simulink model "Caster_4_Whl_Hill"  (R2026a)
settings: Solver=ode23t  StopTime=2.5  FixedStep=1e-3  MaxStep=0.01  RelTol=1e-4  AbsTol=1e-5  EnableMultiTasking=on
StartFcn:
  | tic;
StopFcn:
  | Elapsed_Sim_Time = toc;
  | disp(['Elapsed Sim Time = ' num2str(Elapsed_Sim_Time)]);
model workspace (MATLAB code in the model file):
  | whl.rad = 0.02;
  | whl.thickness = 0.005;
  | 
  | axle.length = 0.2;
  | axle.radius = 0.005;
  | platform.width = 0.1;
  | platform.length = 0.15;
  | platform.thickness = 0.005;
  | platform.offset = 0.05;
  | 
  | caster_axis.rad = 0.005;
  | caster_axis.length = 0.03;
  | 
  | bumper.rad = platform.offset+whl.rad;
  | 
  | 
  | 
  | table.length = 0.5;
  | table.thickness = 0.01;
  | tableWhl.contact.k = 1e3;
  | tableWhl.contact.b = 1e2;
  | 
  | steel.density = 8000; %kg/m^3
  | 
  | start_pos.x = -0.2;
  | start_pos.y = 0.2;
  | 
  | l_whl_trq = [0 0 0 0.5 0 0 0 -0.5 1.0 0 0 0 -1.0 0.5 0 0 0 -0.5 -1.5 0 0 0 1.5].'*0.00005;
  | r_whl_trq = [0 0 0 2.0 0 0 0 -2.0 1.0 0 0 0 -1.0 1.0 0 0 0 -1.0 -1.5 0 0 0 1.5].'*0.00005;
  | 
  | l_whl_trq = [-0.45 0 -0.1 0 0]*7.5e-5*100;
  | r_whl_trq = [-0.45 0 -0.1 0 0]*7.5e-5*100;
  | 
  | muk = 0.7;
  | mus = 0.5;
  | vth =1e-2;
  | 
  | % Floor dimensions
  | flr1_len = 1;
  | flr1_wid = 0.5;
  | flr1_dep = 0.01;
  | flr1_ang = 0;  % deg, rel to world
  | 
  | flr2_len = flr1_len/8;
  | flr2_wid = flr1_wid;
  | flr2_dep = flr1_dep;
  | flr2_ang = 10; % deg, rel to World
  | 
  | flr3_len = flr1_len/3;
  | flr3_wid = flr1_wid;
  | flr3_dep = flr1_dep;
  | flr3_ang = 0;  % deg, rel to World
  | 
  | % Visualize Surfaces
  | flr_dep_pcnt = 0.1;  %(0-1)
  | flr_clr = [1 1 1]*0.95;
undefined symbols (not defined in the file or in its folder): X, Y, Z
libraries: sm_lib x43, Contact_Forces_Lib x16, nesl_utility x5, Parts_Lib x4, simulink x2
(part 2 of 2)

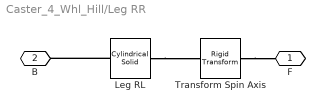
== system Caster_4_Whl_Hill/Leg RR ==
  Leg RL : sm_lib/Body Elements/Cylindrical Solid  CylinderRadius=caster_axis.rad  CylinderRadiusUnits=m  CylinderLength=caster_axis.length  CylinderLengthUnits=m  ExportEntireGeometry=off  InertiaType=CalculateFromGeometry  BasedOnType=Density  Density=1000  DensityUnits=kg/m^3  Mass=1  MassUnits=kg  CenterOfMass=[0 0 0]  CenterOfMassUnits=m  MomentsOfInertia=[1 1 1]  MomentsOfInertiaUnits=kg*m^2  ProductsOfInertia=[0 0 0]  ProductsOfInertiaUnits=kg*m^2  GraphicType=FromGeometry  MarkerShape=Sphere  MarkerSize=10  GraphicVisPropType=SimpleVisualProperties  GraphicDiffuseColor=[0.5 0.5 0.5]  GraphicOpacity=1.0  GraphicSpecularColor=[0.5 0.5 0.5 1.0]  GraphicAmbientColor=[0.15 0.15 0.15 1.0]  GraphicEmissiveColor=[0.0 0.0 0.0 1.0]  GraphicShininess=75  DoExposeReferenceFrame=off  SerializedFrames=<Frames><Frame><Id>Frame1</Id><Value><Name>B</Name><Origin><Source>GeometricFeature</Source><FeatureName>top surface</FeatureName></Origin><PrimaryAxis><DefinedDirection>+Z</DefinedDirection><Source>ReferenceFrame</Source><SourceDirection>+Z</SourceDirection><FeatureName></FeatureName></PrimaryAxis><SecondaryAxis><DefinedDirection>+X</DefinedDirection><Source>ReferenceFrame</Source><SourceDirection>+X</SourceDirection><FeatureName></FeatureName></SecondaryAxis></Value></Frame><Frame><Id>Frame2</Id><Value><Name>F</Name><Origin><Source>GeometricFeature</Source><FeatureName>bottom surface</FeatureName></Origin><PrimaryAxis><DefinedDirection>+Z</DefinedDirection><Source>ReferenceFrame</Source><SourceDirection>+Z</SourceDirection><FeatureName></FeatureName></PrimaryAxis><SecondaryAxis><DefinedDirection>+X</DefinedDirection><Source>ReferenceFrame</Source><SourceDirection>+X</SourceDirection><FeatureName></FeatureName></SecondaryAxis></Value></Frame></Frames>
  Transform Spin Axis : sm_lib/Frames and Transforms/Rigid Transform  RotationMethod=StandardAxis  FollAlignAxisA=+X  BaseAlignAxisA=+Y  FollAlignAxisB=+Y  BaseAlignAxisB=+Z  RotationStandardAxis=+X  RotationAngle=-90  RotationAngleUnits=deg  RotationArbitraryAxis=[0 0 1]  RotationSequenceAxes=FollowerAxes  RotationSequence=XYX  RotationSequenceAngles=[0 0 0]  RotationSequenceAnglesUnits=deg  RotationMatrix=[1 0 0; 0 1 0; 0 0 1]  Quaternion=[1 0 0 0]  TranslationMethod=None  TranslationCartesianOffset=[0 0 0]  TranslationCartesianOffsetUnits=m  TranslationStandardAxis=+Z  TranslationStandardOffset=0  TranslationStandardOffsetUnits=m  TranslationROffset=0  TranslationROffsetUnits=m  TranslationThetaOffset=0  TranslationThetaOffsetUnits=deg  TranslationZOffset=0  TranslationZOffsetUnits=m
  F : PMIOPort  Side=Right
  B : PMIOPort  Port=2  Side=Left
  connections:
  Leg RL/RConn1 -- Transform Spin Axis/LConn1
  Transform Spin Axis/RConn1 -- F/RConn1
  Leg RL/LConn1 -- B/RConn1

== system Caster_4_Whl_Hill/MotorL ==
  Rate Transition : RateTransition
  Repeating Sequence Stair : simulink/Sources/Repeating Sequence Stair  OutValues=l_whl_trq  tsamp=0.7  OutMin=[]  OutMax=[]  OutDataTypeStr=double  OutputDataTypeScalingMode=double  OutDataType=fixdt(0,8)  ConRadixGroup=Best Precision: Vector-wise  OutScaling=2^-12
  Simulink-PS Converter1 : nesl_utility/Simulink-PS Converter  PhysicalDomain=network_engine_domain  SubClassName=ps_input  LeftPortType=input  RightPortType=output  PseudoPeriodic=off  Frequencies=[]  NoiseDistribution=none  NoiseParameters=[]  Unit=1  AffineConversion=off  FilteringAndDerivatives=filter  SimscapeFilterOrder=2  InputFilterTimeConstant=0.005  UdotUserProvided=1
  trq : PMIOPort  Side=Right
  wires:
  Repeating Sequence Stair/1 -> Rate Transition/1
  Rate Transition/1 -> Simulink-PS Converter1/1
  connections:
  trq/RConn1 -- Simulink-PS Converter1/RConn1

== system Caster_4_Whl_Hill/MotorR ==
  Rate Transition : RateTransition
  Repeating Sequence Stair : simulink/Sources/Repeating Sequence Stair  OutValues=r_whl_trq  tsamp=0.7  OutMin=[]  OutMax=[]  OutDataTypeStr=double  OutputDataTypeScalingMode=double  OutDataType=fixdt(0,8)  ConRadixGroup=Best Precision: Vector-wise  OutScaling=2^-12
  Simulink-PS Converter : nesl_utility/Simulink-PS Converter  PhysicalDomain=network_engine_domain  SubClassName=ps_input  LeftPortType=input  RightPortType=output  PseudoPeriodic=off  Frequencies=[]  NoiseDistribution=none  NoiseParameters=[]  Unit=1  AffineConversion=off  FilteringAndDerivatives=filter  SimscapeFilterOrder=2  InputFilterTimeConstant=0.005  UdotUserProvided=1
  trq : PMIOPort  Side=Right
  wires:
  Repeating Sequence Stair/1 -> Rate Transition/1
  Rate Transition/1 -> Simulink-PS Converter/1
  connections:
  Simulink-PS Converter/RConn1 -- trq/RConn1

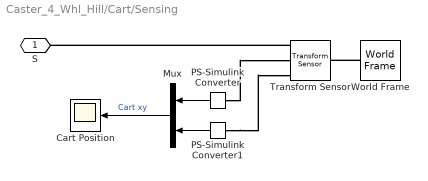
== system Caster_4_Whl_Hill/Cart/Sensing ==
  Cart Position : Scope
      settings: ActiveDisplayYMinimum=-0.86321  ActiveDisplayYMaximum=0.10356  DataLoggingSaveFormat=Array
  Mux : Mux  Inputs=2
  PS-Simulink Converter : nesl_utility/PS-Simulink Converter  PhysicalDomain=network_engine_domain  SubClassName=ps_output  LeftPortType=input  RightPortType=output  PseudoPeriodic=off  Frequencies=[]  VectorFormat=1-D array  Unit=m  AffineConversion=off
  PS-Simulink Converter1 : nesl_utility/PS-Simulink Converter  PhysicalDomain=network_engine_domain  SubClassName=ps_output  LeftPortType=input  RightPortType=output  PseudoPeriodic=off  Frequencies=[]  VectorFormat=1-D array  Unit=m  AffineConversion=off
  Transform Sensor : sm_lib/Frames and Transforms/Transform Sensor  MeasurementFrame=World  RotationSequence=XYX  SenseAngle=off  SenseAxis=off  SenseQ=off  SenseR=off  SenseRotationSequence=off  SenseOmegaX=off  SenseOmegaY=off  SenseOmegaZ=off  SenseOmega=off  SenseQDot=off  SenseRDot=off  SenseRotationSequenceDot=off  SenseAlphaX=off  SenseAlphaY=off  SenseAlphaZ=off  SenseAlpha=off  SenseQDDot=off  SenseRDDot=off  SenseX=on  SenseY=off  SenseZ=on  SenseXYZ=off  SenseRad=off  SenseAzim=off  SenseDist=off  SenseInc=off  SenseXDot=off  SenseYDot=off  SenseZDot=off  SenseXYZDot=off  SenseRadDot=off  SenseAzimDot=off  SenseDistDot=off  SenseIncDot=off  SenseXDDot=off  SenseYDDot=off  SenseZDDot=off  SenseXYZDDot=off  SenseRadDDot=off  SenseAzimDDot=off  SenseDistDDot=off  SenseIncDDot=off
  World Frame : sm_lib/Frames and Transforms/World Frame
  S : PMIOPort  Side=Left
  wires:
  PS-Simulink Converter/1 -> Mux/1
  PS-Simulink Converter1/1 -> Mux/2
  Mux/1 -> Cart Position/1  "Cart xy"
  connections:
  PS-Simulink Converter/LConn1 -- Transform Sensor/RConn2
  World Frame/RConn1 -- Transform Sensor/LConn1
  Transform Sensor/RConn1 -- S/RConn1
  PS-Simulink Converter1/LConn1 -- Transform Sensor/RConn3

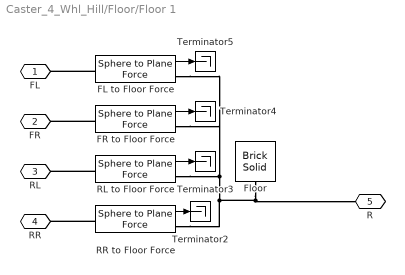
== system Caster_4_Whl_Hill/Floor/Floor 1 ==
  FL to Floor Force : Contact_Forces_Lib/3D/Sphere to Plane Force  sphere_rad=whl.rad  plane_lenx=flr1_len  plane_leny=flr1_wid  plane_depth=flr1_dep/2  force_law=Linear  k_contact=tableWhl.contact.k  b_contact=tableWhl.contact.b  pen_full_damp_F=1e-4  pen_exponent=1  custom_param_1=1  custom_param_2=1  friction_law=Stick-Slip Continuous  mu_kinetic=muk  mu_static=mus  v_thr=vth  vis_on=off  vis_opc_en=0  vis_len_plaBz=flr1_dep*flr_dep_pcnt  vis_clr=[0.9 0.2 0.2]  vis_opc=0.7
  FR to Floor Force : Contact_Forces_Lib/3D/Sphere to Plane Force  sphere_rad=whl.rad  plane_lenx=flr1_len  plane_leny=flr1_wid  plane_depth=flr1_dep/2  force_law=Linear  k_contact=tableWhl.contact.k  b_contact=tableWhl.contact.b  pen_full_damp_F=1e-4  pen_exponent=1  custom_param_1=1  custom_param_2=1  friction_law=Stick-Slip Continuous  mu_kinetic=muk  mu_static=mus  v_thr=vth  vis_on=off  vis_opc_en=0  vis_len_plaBz=flr1_dep*flr_dep_pcnt  vis_clr=[0.9 0.2 0.2]  vis_opc=0.7
  Floor : sm_lib/Body Elements/Brick Solid  BrickDimensions=[flr1_len flr1_wid flr1_dep]  BrickDimensionsUnits=m  ExportEntireGeometry=off  InertiaType=CalculateFromGeometry  BasedOnType=Density  Density=1000  DensityUnits=kg/m^3  Mass=1  MassUnits=kg  CenterOfMass=[0 0 0]  CenterOfMassUnits=m  MomentsOfInertia=[1 1 1]  MomentsOfInertiaUnits=kg*m^2  ProductsOfInertia=[0 0 0]  ProductsOfInertiaUnits=kg*m^2  GraphicType=FromGeometry  MarkerShape=Sphere  MarkerSize=10  GraphicVisPropType=SimpleVisualProperties  GraphicDiffuseColor=flr_clr  GraphicOpacity=1.0  GraphicSpecularColor=[0.5 0.5 0.5 1.0]  GraphicAmbientColor=[0.15 0.15 0.15 1.0]  GraphicEmissiveColor=[0.0 0.0 0.0 1.0]  GraphicShininess=75  DoExposeReferenceFrame=on  SerializedFrames=<Frames/>
  RL to Floor Force : Contact_Forces_Lib/3D/Sphere to Plane Force  sphere_rad=whl.rad  plane_lenx=flr1_len  plane_leny=flr1_wid  plane_depth=flr1_dep/2  force_law=Linear  k_contact=tableWhl.contact.k  b_contact=tableWhl.contact.b  pen_full_damp_F=1e-4  pen_exponent=1  custom_param_1=1  custom_param_2=1  friction_law=Stick-Slip Continuous  mu_kinetic=muk  mu_static=mus  v_thr=vth  vis_on=off  vis_opc_en=0  vis_len_plaBz=flr1_dep*flr_dep_pcnt  vis_clr=[0.9 0.2 0.2]  vis_opc=0.7
  RR to Floor Force : Contact_Forces_Lib/3D/Sphere to Plane Force  sphere_rad=whl.rad  plane_lenx=flr1_len  plane_leny=flr1_wid  plane_depth=flr1_dep/2  force_law=Linear  k_contact=tableWhl.contact.k  b_contact=tableWhl.contact.b  pen_full_damp_F=1e-4  pen_exponent=1  custom_param_1=1  custom_param_2=1  friction_law=Stick-Slip Continuous  mu_kinetic=muk  mu_static=mus  v_thr=vth  vis_on=off  vis_opc_en=0  vis_len_plaBz=flr1_dep*flr_dep_pcnt  vis_clr=[0.9 0.2 0.2]  vis_opc=0.7
  Terminator{2..5} (4 alike) : Terminator
  FL : PMIOPort  Side=Left
  FR : PMIOPort  Port=2  Side=Left
  RL : PMIOPort  Port=3  Side=Left
  RR : PMIOPort  Port=4  Side=Left
  R : PMIOPort  Port=5  Side=Right
  wires:
  FR to Floor Force/1 -> Terminator4/1
  FL to Floor Force/1 -> Terminator5/1
  RL to Floor Force/1 -> Terminator3/1
  RR to Floor Force/1 -> Terminator2/1
  connections:
  Floor/RConn1 -- R/RConn1 -- RR to Floor Force/RConn1 -- RL to Floor Force/RConn1 -- FR to Floor Force/RConn1 -- FL to Floor Force/RConn1
  FR to Floor Force/LConn1 -- FR/RConn1
  RR to Floor Force/LConn1 -- RR/RConn1
  RL to Floor Force/LConn1 -- RL/RConn1
  FL to Floor Force/LConn1 -- FL/RConn1

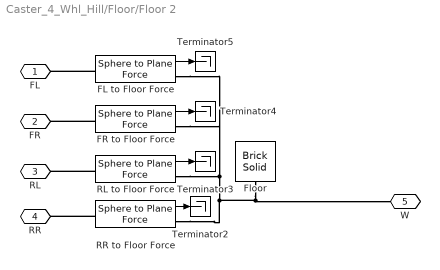
== system Caster_4_Whl_Hill/Floor/Floor 2 ==
  FL to Floor Force : Contact_Forces_Lib/3D/Sphere to Plane Force  sphere_rad=whl.rad  plane_lenx=flr2_len  plane_leny=flr2_wid  plane_depth=flr2_dep/2  force_law=Linear  k_contact=tableWhl.contact.k  b_contact=tableWhl.contact.b  pen_full_damp_F=1e-4  pen_exponent=1  custom_param_1=1  custom_param_2=1  friction_law=Stick-Slip Continuous  mu_kinetic=muk  mu_static=mus  v_thr=vth  vis_on=off  vis_opc_en=0  vis_len_plaBz=flr2_dep*flr_dep_pcnt  vis_clr=[0.9 0.2 0.2]  vis_opc=0.7
  FR to Floor Force : Contact_Forces_Lib/3D/Sphere to Plane Force  sphere_rad=whl.rad  plane_lenx=flr2_len  plane_leny=flr2_wid  plane_depth=flr2_dep/2  force_law=Linear  k_contact=tableWhl.contact.k  b_contact=tableWhl.contact.b  pen_full_damp_F=1e-4  pen_exponent=1  custom_param_1=1  custom_param_2=1  friction_law=Stick-Slip Continuous  mu_kinetic=muk  mu_static=mus  v_thr=vth  vis_on=off  vis_opc_en=0  vis_len_plaBz=flr2_dep*flr_dep_pcnt  vis_clr=[0.9 0.2 0.2]  vis_opc=0.7
  Floor : sm_lib/Body Elements/Brick Solid  BrickDimensions=[flr2_len flr2_wid flr2_dep]  BrickDimensionsUnits=m  ExportEntireGeometry=off  InertiaType=CalculateFromGeometry  BasedOnType=Density  Density=1000  DensityUnits=kg/m^3  Mass=1  MassUnits=kg  CenterOfMass=[0 0 0]  CenterOfMassUnits=m  MomentsOfInertia=[1 1 1]  MomentsOfInertiaUnits=kg*m^2  ProductsOfInertia=[0 0 0]  ProductsOfInertiaUnits=kg*m^2  GraphicType=FromGeometry  MarkerShape=Sphere  MarkerSize=10  GraphicVisPropType=SimpleVisualProperties  GraphicDiffuseColor=flr_clr  GraphicOpacity=1.0  GraphicSpecularColor=[0.5 0.5 0.5 1.0]  GraphicAmbientColor=[0.15 0.15 0.15 1.0]  GraphicEmissiveColor=[0.0 0.0 0.0 1.0]  GraphicShininess=75  DoExposeReferenceFrame=on  SerializedFrames=<Frames/>
  RL to Floor Force : Contact_Forces_Lib/3D/Sphere to Plane Force  sphere_rad=whl.rad  plane_lenx=flr2_len  plane_leny=flr2_wid  plane_depth=flr2_dep/2  force_law=Linear  k_contact=tableWhl.contact.k  b_contact=tableWhl.contact.b  pen_full_damp_F=1e-4  pen_exponent=1  custom_param_1=1  custom_param_2=1  friction_law=Stick-Slip Continuous  mu_kinetic=muk  mu_static=mus  v_thr=vth  vis_on=off  vis_opc_en=0  vis_len_plaBz=flr2_dep*flr_dep_pcnt  vis_clr=[0.9 0.2 0.2]  vis_opc=0.7
  RR to Floor Force : Contact_Forces_Lib/3D/Sphere to Plane Force  sphere_rad=whl.rad  plane_lenx=flr2_len  plane_leny=flr2_wid  plane_depth=flr2_dep/2  force_law=Linear  k_contact=tableWhl.contact.k  b_contact=tableWhl.contact.b  pen_full_damp_F=1e-4  pen_exponent=1  custom_param_1=1  custom_param_2=1  friction_law=Stick-Slip Continuous  mu_kinetic=muk  mu_static=mus  v_thr=vth  vis_on=off  vis_opc_en=0  vis_len_plaBz=flr2_dep*flr_dep_pcnt  vis_clr=[0.9 0.2 0.2]  vis_opc=0.7
  Terminator{2..5} (4 alike) : Terminator
  FL : PMIOPort  Side=Left
  FR : PMIOPort  Port=2  Side=Left
  RL : PMIOPort  Port=3  Side=Left
  RR : PMIOPort  Port=4  Side=Left
  W : PMIOPort  Port=5  Side=Right
  wires:
  RR to Floor Force/1 -> Terminator2/1
  RL to Floor Force/1 -> Terminator3/1
  FL to Floor Force/1 -> Terminator5/1
  FR to Floor Force/1 -> Terminator4/1
  connections:
  FL to Floor Force/LConn1 -- FL/RConn1
  RL to Floor Force/LConn1 -- RL/RConn1
  RR to Floor Force/LConn1 -- RR/RConn1
  FR to Floor Force/LConn1 -- FR/RConn1
  Floor/RConn1 -- W/RConn1 -- RR to Floor Force/RConn1 -- FL to Floor Force/RConn1 -- FR to Floor Force/RConn1 -- RL to Floor Force/RConn1

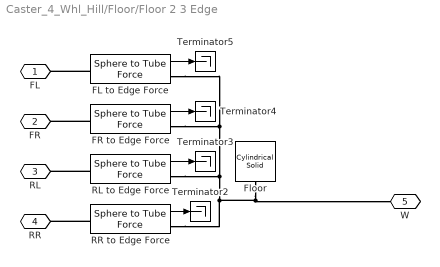
== system Caster_4_Whl_Hill/Floor/Floor 2 3 Edge ==
  FL to Edge Force : Contact_Forces_Lib/3D/Sphere to Tube Force  radius_sphere=whl.rad  radius_tube=flr2_dep/2*(1-0.1)  d_tube=flr2_dep/2*(2*0.1)  l_tube=flr2_wid  active_angle=[-flr2_ang 0]  force_law=Linear  k_contact=tableWhl.contact.k  b_contact=tableWhl.contact.b  pen_full_damp_F=1e-4  pen_exponent=1  custom_param_1=1  custom_param_2=1  friction_law=Stick-Slip Continuous  mu_kinetic=muk  mu_static=mus  v_thr=vth  vis_on=off  vis_opc_en=0  vis_len_tubBx=flr2_dep*flr_dep_pcnt  vis_clr=[0.9 0.2 0.2]  vis_opc=0.7
      settings: SourceProductName=Simscape Multibody Contact Forces Library
  FR to Edge Force : Contact_Forces_Lib/3D/Sphere to Tube Force  radius_sphere=whl.rad  radius_tube=flr2_dep/2*(1-0.1)  d_tube=flr2_dep/2*(2*0.1)  l_tube=flr2_wid  active_angle=[-flr2_ang 0]  force_law=Linear  k_contact=tableWhl.contact.k  b_contact=tableWhl.contact.b  pen_full_damp_F=1e-4  pen_exponent=1  custom_param_1=1  custom_param_2=1  friction_law=Stick-Slip Continuous  mu_kinetic=muk  mu_static=mus  v_thr=vth  vis_on=off  vis_opc_en=0  vis_len_tubBx=flr2_dep*flr_dep_pcnt  vis_clr=[0.9 0.2 0.2]  vis_opc=0.7
      settings: SourceProductName=Simscape Multibody Contact Forces Library
  Floor : sm_lib/Body Elements/Cylindrical Solid  CylinderRadius=flr2_dep/2  CylinderRadiusUnits=m  CylinderLength=flr2_wid  CylinderLengthUnits=m  ExportEntireGeometry=off  InertiaType=CalculateFromGeometry  BasedOnType=Density  Density=1000  DensityUnits=kg/m^3  Mass=1  MassUnits=kg  CenterOfMass=[0 0 0]  CenterOfMassUnits=m  MomentsOfInertia=[1 1 1]  MomentsOfInertiaUnits=kg*m^2  ProductsOfInertia=[0 0 0]  ProductsOfInertiaUnits=kg*m^2  GraphicType=FromGeometry  MarkerShape=Sphere  MarkerSize=10  GraphicVisPropType=SimpleVisualProperties  GraphicDiffuseColor=flr_clr  GraphicOpacity=1.0  GraphicSpecularColor=[0.5 0.5 0.5 1.0]  GraphicAmbientColor=[0.15 0.15 0.15 1.0]  GraphicEmissiveColor=[0.0 0.0 0.0 1.0]  GraphicShininess=75  DoExposeReferenceFrame=on  SerializedFrames=<Frames/>
  RL to Edge Force : Contact_Forces_Lib/3D/Sphere to Tube Force  radius_sphere=whl.rad  radius_tube=flr2_dep/2*(1-0.1)  d_tube=flr2_dep/2*(2*0.1)  l_tube=flr2_wid  active_angle=[-flr2_ang 0]  force_law=Linear  k_contact=tableWhl.contact.k  b_contact=tableWhl.contact.b  pen_full_damp_F=1e-4  pen_exponent=1  custom_param_1=1  custom_param_2=1  friction_law=Stick-Slip Continuous  mu_kinetic=muk  mu_static=mus  v_thr=vth  vis_on=off  vis_opc_en=0  vis_len_tubBx=flr2_dep*flr_dep_pcnt  vis_clr=[0.9 0.2 0.2]  vis_opc=0.7
      settings: SourceProductName=Simscape Multibody Contact Forces Library
  RR to Edge Force : Contact_Forces_Lib/3D/Sphere to Tube Force  radius_sphere=whl.rad  radius_tube=flr2_dep/2*(1-0.1)  d_tube=flr2_dep/2*(2*0.1)  l_tube=flr2_wid  active_angle=[-flr2_ang 0]  force_law=Linear  k_contact=tableWhl.contact.k  b_contact=tableWhl.contact.b  pen_full_damp_F=1e-4  pen_exponent=1  custom_param_1=1  custom_param_2=1  friction_law=Stick-Slip Continuous  mu_kinetic=muk  mu_static=mus  v_thr=vth  vis_on=off  vis_opc_en=0  vis_len_tubBx=flr2_dep*flr_dep_pcnt  vis_clr=[0.9 0.2 0.2]  vis_opc=0.7
      settings: SourceProductName=Simscape Multibody Contact Forces Library
  Terminator{2..5} (4 alike) : Terminator
  FL : PMIOPort  Side=Left
  FR : PMIOPort  Port=2  Side=Left
  RL : PMIOPort  Port=3  Side=Left
  RR : PMIOPort  Port=4  Side=Left
  W : PMIOPort  Port=5  Side=Right
  wires:
  FR to Edge Force/1 -> Terminator4/1
  FL to Edge Force/1 -> Terminator5/1
  RL to Edge Force/1 -> Terminator3/1
  RR to Edge Force/1 -> Terminator2/1
  connections:
  RL to Edge Force/RConn1 -- FR to Edge Force/RConn1 -- FL to Edge Force/RConn1 -- RR to Edge Force/RConn1 -- W/RConn1 -- Floor/RConn1
  FR to Edge Force/LConn1 -- FR/RConn1
  RR to Edge Force/LConn1 -- RR/RConn1
  RL to Edge Force/LConn1 -- RL/RConn1
  FL to Edge Force/LConn1 -- FL/RConn1

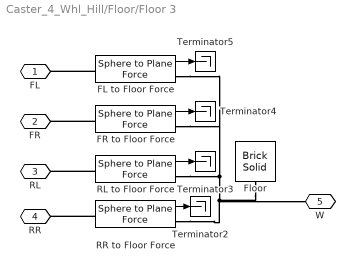
== system Caster_4_Whl_Hill/Floor/Floor 3 ==
  FL to Floor Force : Contact_Forces_Lib/3D/Sphere to Plane Force  sphere_rad=whl.rad  plane_lenx=flr3_len  plane_leny=flr3_wid  plane_depth=flr3_dep/2  force_law=Linear  k_contact=tableWhl.contact.k  b_contact=tableWhl.contact.b  pen_full_damp_F=1e-4  pen_exponent=1  custom_param_1=1  custom_param_2=1  friction_law=Stick-Slip Continuous  mu_kinetic=muk  mu_static=mus  v_thr=vth  vis_on=off  vis_opc_en=0  vis_len_plaBz=flr3_dep*flr_dep_pcnt  vis_clr=[0.9 0.2 0.2]  vis_opc=0.7
  FR to Floor Force : Contact_Forces_Lib/3D/Sphere to Plane Force  sphere_rad=whl.rad  plane_lenx=flr3_len  plane_leny=flr3_wid  plane_depth=flr3_dep/2  force_law=Linear  k_contact=tableWhl.contact.k  b_contact=tableWhl.contact.b  pen_full_damp_F=1e-4  pen_exponent=1  custom_param_1=1  custom_param_2=1  friction_law=Stick-Slip Continuous  mu_kinetic=muk  mu_static=mus  v_thr=vth  vis_on=off  vis_opc_en=0  vis_len_plaBz=flr3_dep*flr_dep_pcnt  vis_clr=[0.9 0.2 0.2]  vis_opc=0.7
  Floor : sm_lib/Body Elements/Brick Solid  BrickDimensions=[flr3_len flr3_wid flr3_dep]  BrickDimensionsUnits=m  ExportEntireGeometry=off  InertiaType=CalculateFromGeometry  BasedOnType=Density  Density=1000  DensityUnits=kg/m^3  Mass=1  MassUnits=kg  CenterOfMass=[0 0 0]  CenterOfMassUnits=m  MomentsOfInertia=[1 1 1]  MomentsOfInertiaUnits=kg*m^2  ProductsOfInertia=[0 0 0]  ProductsOfInertiaUnits=kg*m^2  GraphicType=FromGeometry  MarkerShape=Sphere  MarkerSize=10  GraphicVisPropType=SimpleVisualProperties  GraphicDiffuseColor=flr_clr  GraphicOpacity=1.0  GraphicSpecularColor=[0.5 0.5 0.5 1.0]  GraphicAmbientColor=[0.15 0.15 0.15 1.0]  GraphicEmissiveColor=[0.0 0.0 0.0 1.0]  GraphicShininess=75  DoExposeReferenceFrame=on  SerializedFrames=<Frames/>
  RL to Floor Force : Contact_Forces_Lib/3D/Sphere to Plane Force  sphere_rad=whl.rad  plane_lenx=flr3_len  plane_leny=flr3_wid  plane_depth=flr3_dep/2  force_law=Linear  k_contact=tableWhl.contact.k  b_contact=tableWhl.contact.b  pen_full_damp_F=1e-4  pen_exponent=1  custom_param_1=1  custom_param_2=1  friction_law=Stick-Slip Continuous  mu_kinetic=muk  mu_static=mus  v_thr=vth  vis_on=off  vis_opc_en=0  vis_len_plaBz=flr3_dep*flr_dep_pcnt  vis_clr=[0.9 0.2 0.2]  vis_opc=0.7
  RR to Floor Force : Contact_Forces_Lib/3D/Sphere to Plane Force  sphere_rad=whl.rad  plane_lenx=flr3_len  plane_leny=flr3_wid  plane_depth=flr3_dep/2  force_law=Linear  k_contact=tableWhl.contact.k  b_contact=tableWhl.contact.b  pen_full_damp_F=1e-4  pen_exponent=1  custom_param_1=1  custom_param_2=1  friction_law=Stick-Slip Continuous  mu_kinetic=muk  mu_static=mus  v_thr=vth  vis_on=off  vis_opc_en=0  vis_len_plaBz=flr3_dep*flr_dep_pcnt  vis_clr=[0.9 0.2 0.2]  vis_opc=0.7
  Terminator{2..5} (4 alike) : Terminator
  FL : PMIOPort  Side=Left
  FR : PMIOPort  Port=2  Side=Left
  RL : PMIOPort  Port=3  Side=Left
  RR : PMIOPort  Port=4  Side=Left
  W : PMIOPort  Port=5  Side=Right
  wires:
  FR to Floor Force/1 -> Terminator4/1
  FL to Floor Force/1 -> Terminator5/1
  RL to Floor Force/1 -> Terminator3/1
  RR to Floor Force/1 -> Terminator2/1
  connections:
  FR to Floor Force/LConn1 -- FR/RConn1
  RR to Floor Force/LConn1 -- RR/RConn1
  RL to Floor Force/LConn1 -- RL/RConn1
  FL to Floor Force/LConn1 -- FL/RConn1
  RL to Floor Force/RConn1 -- RR to Floor Force/RConn1 -- W/RConn1 -- Floor/RConn1 -- FR to Floor Force/RConn1 -- FL to Floor Force/RConn1

== system Caster_4_Whl_Hill/Floor/Transform Floor 3 ==
  Transform Plane Ref Ctr Floor 3 : sm_lib/Frames and Transforms/Rigid Transform  RotationMethod=None  FollAlignAxisA=+X  BaseAlignAxisA=+Y  FollAlignAxisB=+Y  BaseAlignAxisB=+Z  RotationStandardAxis=+Y  RotationAngle=-10  RotationAngleUnits=deg  RotationArbitraryAxis=[0 0 1]  RotationSequenceAxes=FollowerAxes  RotationSequence=XYX  RotationSequenceAngles=[0 0 0]  RotationSequenceAnglesUnits=deg  RotationMatrix=[1 0 0; 0 1 0; 0 0 1]  Quaternion=[1 0 0 0]  TranslationMethod=Cartesian  TranslationCartesianOffset=[flr3_len/2 0 0]  TranslationCartesianOffsetUnits=m  TranslationStandardAxis=+Z  TranslationStandardOffset=0  TranslationStandardOffsetUnits=m  TranslationROffset=0  TranslationROffsetUnits=m  TranslationThetaOffset=0  TranslationThetaOffsetUnits=deg  TranslationZOffset=0  TranslationZOffsetUnits=m
  Transform Plane Ref Floor 1 End : sm_lib/Frames and Transforms/Rigid Transform  RotationMethod=None  FollAlignAxisA=+X  BaseAlignAxisA=+Y  FollAlignAxisB=+Y  BaseAlignAxisB=+Z  RotationStandardAxis=+Y  RotationAngle=-10  RotationAngleUnits=deg  RotationArbitraryAxis=[0 0 1]  RotationSequenceAxes=FollowerAxes  RotationSequence=XYX  RotationSequenceAngles=[0 0 0]  RotationSequenceAnglesUnits=deg  RotationMatrix=[1 0 0; 0 1 0; 0 0 1]  Quaternion=[1 0 0 0]  TranslationMethod=Cartesian  TranslationCartesianOffset=[cosd(flr2_ang) 0 sind(flr2_ang)]*flr2_len  TranslationCartesianOffsetUnits=m  TranslationStandardAxis=+Z  TranslationStandardOffset=0  TranslationStandardOffsetUnits=m  TranslationROffset=0  TranslationROffsetUnits=m  TranslationThetaOffset=0  TranslationThetaOffsetUnits=deg  TranslationZOffset=0  TranslationZOffsetUnits=m
  F : PMIOPort  Side=Right
  B : PMIOPort  Port=2  Side=Left
  connections:
  Transform Plane Ref Floor 1 End/RConn1 -- Transform Plane Ref Ctr Floor 3/LConn1
  Transform Plane Ref Floor 1 End/LConn1 -- B/RConn1
  F/RConn1 -- Transform Plane Ref Ctr Floor 3/RConn1
